simulink model "sim_ADRC_1link_arm"  (R2020b)
settings: Solver=FixedStepAuto  StartTime=0.0  StopTime=2  FixedStep=0.0001  RelTol=1e-3
values from neighbouring files (symbols this model uses):
  A_ex = [0 1 0; 0 0 1; 0 0 0 ]    [ADRC_1link_arm.m]
  B_ex = [0; B(2); 0]    [ADRC_1link_arm.m]
  b_inv = 1/B(2)    [ADRC_1link_arm.m]
  C_ex = [1 0 0]    [ADRC_1link_arm.m]
  c_theta = 0.2    [ADRC_1link_arm.m]
  dtheta_ini = 0    [ADRC_1link_arm.m]
  g = 9.8    [ADRC_1link_arm.m]    (also in ADRC_2link_arm.m)
  I = M*l^2/12 + (l/2)^2*M    (= 0.333333333333)    [ADRC_1link_arm.m]
  Kd = F_ctrl(2)    [ADRC_1link_arm.m]
  kd = 40    [ADRC_1link_arm.m]
  Ki = -F_ctrl(n+1)    [ADRC_1link_arm.m]
  Kp = F_ctrl(1)    [ADRC_1link_arm.m]
  kp = 600    [ADRC_1link_arm.m]
  l = 1    [ADRC_1link_arm.m]
  L_ex = [c2;c1;c0]    [ADRC_1link_arm.m]
  M = 1    [ADRC_1link_arm.m]
  theta_ini = pi/4    (= 0.785398163397)    [ADRC_1link_arm.m]
settings Model: Creator=s0612  LastModifiedBy=s0612

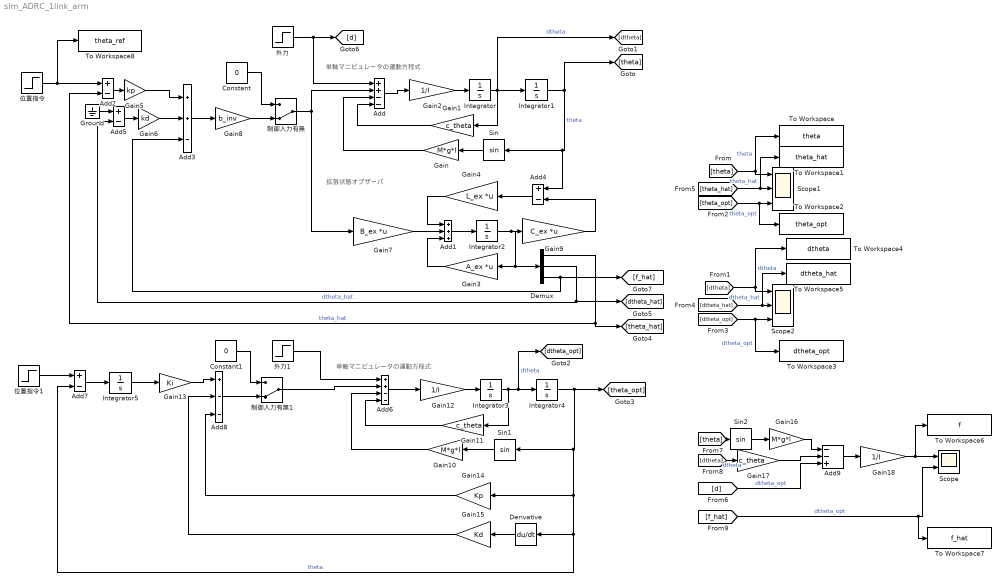
== system sim_ADRC_1link_arm ==
  note: 拡張状態オブザーバ
  note: 単軸マニピュレータの運動方程式
  note: 単軸マニピュレータの運動方程式
  Add : Sum  Inputs=++--
  Add1 : Sum  Inputs=+++
  Add{2,4..5,7} (4 alike) : Sum  Inputs=+-
  Add3 : Sum  Inputs=++-
  Add6 : Sum  Inputs=++--
  Add8 : Sum  Inputs=+--
  Add9 : Sum  Inputs=--+
  Constant : Constant  Value=0
  Constant1 : Constant  Value=0
  Demux : Demux  Outputs=3
  Derivative : Derivative
  Gain : Gain  Gain=M*g*l
  Gain1 : Gain  Gain=c_theta
  Gain10 : Gain  Gain=M*g*l
  Gain11 : Gain  Gain=c_theta
  Gain12 : Gain  Gain=1/I
  Gain13 : Gain  Gain=Ki
  Gain14 : Gain  Gain=Kp
  Gain15 : Gain  Gain=Kd
  Gain16 : Gain  Gain=M*g*l
  Gain17 : Gain  Gain=c_theta
  Gain18 : Gain  Gain=1/I
  Gain2 : Gain  Gain=1/I
  Gain3 : Gain  Gain=A_ex  Multiplication=Matrix(K*u) (u vector)
  Gain4 : Gain  Gain=L_ex  Multiplication=Matrix(K*u) (u vector)
  Gain5 : Gain  Gain=kp
  Gain6 : Gain  Gain=kd
  Gain7 : Gain  Gain=B_ex  Multiplication=Matrix(K*u) (u vector)
  Gain8 : Gain  Gain=b_inv
  Gain9 : Gain  Gain=C_ex  Multiplication=Matrix(K*u) (u vector)
  Ground : Ground
  Integrator : Integrator  InitialCondition=dtheta_ini
  Integrator1 : Integrator  InitialCondition=theta_ini
  Integrator2 : Integrator
  Integrator3 : Integrator  InitialCondition=dtheta_ini
  Integrator4 : Integrator  InitialCondition=theta_ini
  Integrator5 : Integrator
  Scope : Scope  NumInputPorts=2
  Scope1 : Scope  NumInputPorts=3
  Scope2 : Scope  NumInputPorts=3
  Sin : Trigonometry
  Sin1 : Trigonometry
  Sin2 : Trigonometry
  To Workspace : ToWorkspace  VariableName=theta  SaveFormat=Timeseries  SampleTime=-1
  To Workspace1 : ToWorkspace  VariableName=theta_hat  SaveFormat=Timeseries  SampleTime=-1
  To Workspace2 : ToWorkspace  VariableName=theta_opt  SaveFormat=Timeseries  SampleTime=-1
  To Workspace3 : ToWorkspace  VariableName=dtheta_opt  SaveFormat=Timeseries  SampleTime=-1
  To Workspace4 : ToWorkspace  VariableName=dtheta  SaveFormat=Timeseries  SampleTime=-1
  To Workspace5 : ToWorkspace  VariableName=dtheta_hat  SaveFormat=Timeseries  SampleTime=-1
  To Workspace6 : ToWorkspace  VariableName=f  SaveFormat=Timeseries  SampleTime=-1
  To Workspace7 : ToWorkspace  VariableName=f_hat  SaveFormat=Timeseries  SampleTime=-1
  To Workspace8 : ToWorkspace  VariableName=theta_ref  SaveFormat=Timeseries  SampleTime=-1
  位置指令 : Step  Time=0.5  After=pi/2  SampleTime=0
  位置指令1 : Step  Time=0.5  After=pi/2  SampleTime=0
  制御入力有無 : ManualSwitch  CurrentSetting=0
  制御入力有無1 : ManualSwitch  CurrentSetting=0
  外力 : Step  Time=1.5  After=30  SampleTime=0
  外力1 : Step  Time=1.5  After=10  SampleTime=0
  wires:
  Integrator/1 -> [dtheta], Gain1/1, Integrator1/1  "dtheta"
  Integrator1/1 -> Add4/1, Sin/1, [theta]  "theta"
  Add/1 -> Gain2/1
  Sin/1 -> Gain/1
  Gain/1 -> Add/3
  Gain1/1 -> Add/4
  Gain2/1 -> Integrator/1
  制御入力有無/1 -> Add/2, Gain7/1
  Integrator2/1 -> Demux/1, Gain3/1, Gain9/1
  Add1/1 -> Integrator2/1
  Gain3/1 -> Add1/3
  Gain4/1 -> Add1/1
  [theta] -> To Workspace/1, Scope1/1  "theta"
  Demux/1 -> Add2/2, [theta_hat]  "theta_hat"
  位置指令/1 -> To Workspace8/1, Add2/1
  Add2/1 -> Gain5/1
  Gain5/1 -> Add3/1
  Gain6/1 -> Add3/2
  Demux/2 -> Add5/2, [dtheta_hat]  "dtheta_hat"
  Gain7/1 -> Add1/2
  [dtheta] -> To Workspace4/1, Scope2/1  "dtheta"
  Add4/1 -> Gain4/1
  Gain9/1 -> Add4/2
  Add3/1 -> Gain8/1
  Constant/1 -> 制御入力有無/1
  Add5/1 -> Gain6/1
  Demux/3 -> Add3/3, [f_hat]
  Sin1/1 -> Gain10/1
  Gain10/1 -> Add6/3
  制御入力有無1/1 -> Add6/2
  Gain11/1 -> Add6/4
  Gain12/1 -> Integrator3/1
  Integrator4/1 -> [theta_opt], Add7/2, Derivative/1, Gain14/1, Sin1/1  "theta"
  Integrator3/1 -> Gain11/1, [dtheta_opt], Integrator4/1  "dtheta"
  Add6/1 -> Gain12/1
  Add8/1 -> 制御入力有無1/2
  Gain13/1 -> Add8/1
  Gain14/1 -> Add8/3
  位置指令1/1 -> Add7/1
  Add7/1 -> Integrator5/1
  Constant1/1 -> 制御入力有無1/1
  [theta_opt] -> To Workspace2/1, Scope1/3  "theta_opt"
  [dtheta_opt] -> To Workspace3/1, Scope2/3  "dtheta_opt"
  Integrator5/1 -> Gain13/1
  Derivative/1 -> Gain15/1
  Gain15/1 -> Add8/2
  外力/1 -> [d], Add/1
  外力1/1 -> Add6/1
  [dtheta_hat] -> To Workspace5/1, Scope2/2  "dtheta_hat"
  [theta_hat] -> To Workspace1/1, Scope1/2  "theta_hat"
  Ground/1 -> Add5/1
  Sin2/1 -> Gain16/1
  [theta] -> Sin2/1
  [dtheta] -> Gain17/1  "dtheta"
  Gain17/1 -> Add9/2
  Gain16/1 -> Add9/1
  Add9/1 -> Gain18/1
  [d] -> Add9/3  "dtheta_opt"
  Gain18/1 -> To Workspace6/1, Scope/1
  [f_hat] -> To Workspace7/1, Scope/2  "dtheta_opt"
  Gain8/1 -> 制御入力有無/2
